simulink model "Subsystem"  (R2020b)
settings: Solver=VariableStepAuto  StartTime=0.0  StopTime=10.0  RelTol=1e-3
values from neighbouring files (symbols this model uses):
  b = 0.1    [motor_control_model_variables.sldd]    (also in variable_values.mat; variables.mat = 3.5077e-06)
  J = 0.01    [motor_control_model_variables.sldd]    (also in variable_values.mat; variables.mat = 3.2284e-06)
  K = 0.01    [motor_control_model_variables.sldd]    (also in variable_values.mat; variables.mat = 0.0274)
  Kd = 0.15    [motor_control_model_variables.sldd]    (also in variable_values.mat; variables.mat = -0.15)
  Ki = 500.0    [motor_control_model_variables.sldd]    (also in variable_values.mat = 500; variables.mat = -750)
  Kp = 60.0    [motor_control_model_variables.sldd]    (also in variable_values.mat = 20; variables.mat = -20)
  L = 2.75E-6    [motor_control_model_variables.sldd]    (also in variable_values.mat = 0.5; variables.mat = 2.75e-06)
  R = 4.0    [motor_control_model_variables.sldd]    (also in variable_values.mat = 1; variables.mat = 4)
  Ts = 0.01    [motor_control_model_variables.sldd]    (also in variable_values.mat)
settings Model: DataDictionary=motor_control_model_variables.sldd  Creator=DELL  LastModifiedBy=DELL
settings DataIOCC: SaveOutput=off  SaveTime=off

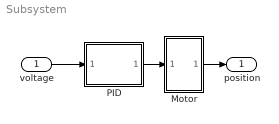
== system Subsystem ==
  voltage : Inport  OutDataTypeStr=double  PortDimensions=1  SampleTime=0
  Motor : Subsystem
  PID : Subsystem
  position : Outport  OutDataTypeStr=double  PortDimensions=1  SampleTime=0
  wires:
  PID/1(Output1) -> Motor/1(In1)
  voltage/1 -> PID/1(Inport)
  Motor/1(Outport) -> position/1

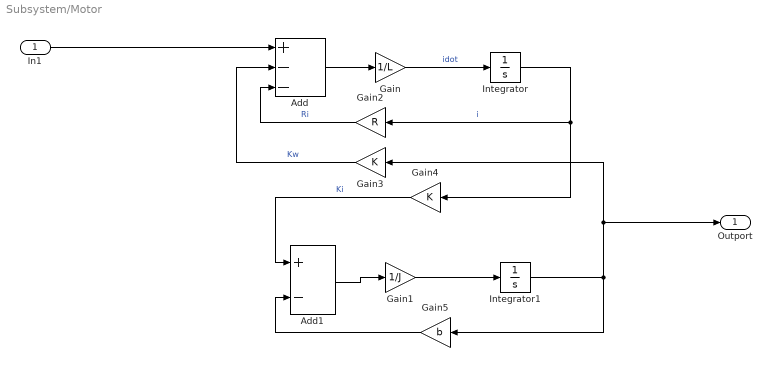
== system Subsystem/Motor ==
  In1 : Inport
  Add : Sum  Inputs=+--
  Add1 : Sum  Inputs=+-
  Gain : Gain  Gain=1/L
  Gain1 : Gain  Gain=1/J
  Gain2 : Gain  Gain=R
  Gain3 : Gain  Gain=K
  Gain4 : Gain  Gain=K
  Gain5 : Gain  Gain=b
  Integrator : Integrator
  Integrator1 : Integrator
  Outport : Outport
  wires:
  Gain5/1 -> Add1/2
  In1/1 -> Add/1
  Gain/1 -> Integrator/1  "idot"
  Gain1/1 -> Integrator1/1
  Gain2/1 -> Add/3  "Ri"
  Add/1 -> Gain/1
  Gain4/1 -> Add1/1  "Ki"
  Gain3/1 -> Add/2  "Kw"
  Add1/1 -> Gain1/1
  Integrator1/1 -> Gain5/1, Gain3/1, Outport/1
  Integrator/1 -> Gain2/1, Gain4/1  "i"

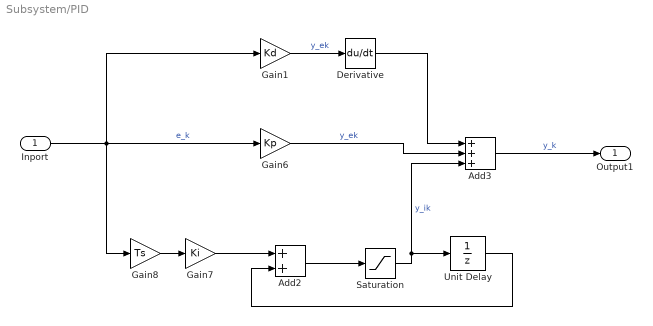
== system Subsystem/PID ==
  Inport : Inport
  Add2 : Sum
  Add3 : Sum  Inputs=+++
  Derivative : Derivative
  Gain1 : Gain  Gain=Kd
  Gain6 : Gain  Gain=Kp
  Gain7 : Gain  Gain=Ki
  Gain8 : Gain  Gain=Ts
  Saturation : Saturate  UpperLimit=1  LowerLimit=-1
  Unit Delay : UnitDelay  SampleTime=-1  HasFrameUpgradeWarning=on
  Output1 : Outport
  wires:
  Derivative/1 -> Add3/1
  Gain1/1 -> Derivative/1  "y_ek"
  Gain7/1 -> Add2/1
  Unit Delay/1 -> Add2/2
  Add3/1 -> Output1/1  "y_k"
  Add2/1 -> Saturation/1
  Saturation/1 -> Add3/3, Unit Delay/1  "y_ik"
  Gain8/1 -> Gain7/1
  Gain6/1 -> Add3/2  "y_ek"
  Inport/1 -> Gain6/1, Gain8/1, Gain1/1  "e_k"
